simulink model "mesh"  (R2015a)
settings: Solver=ode45  StartTime=0.0  StopTime=10.0  RelTol=1e-3
libraries: fl_lib x7, nesl_utility x3
settings Model: SimulationMode=external  Creator=ASUS  LastModifiedBy=ASUS

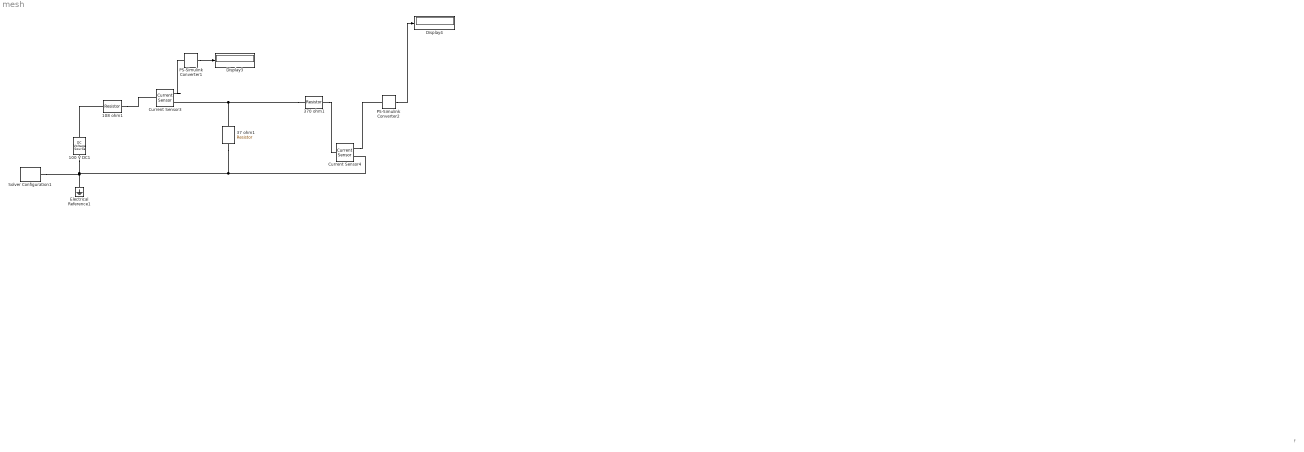
== system mesh ==
  note: f
  " 37 ohm1" : fl_lib/Electrical/Electrical Elements/Resistor  R=37 Ohm  i_specify=off  i_priority=High  i=0 A  v_specify=off  v_priority=High  v=0 V
  100 V DC1 : fl_lib/Electrical/Electrical Sources/DC Voltage Source  v0=100 V
  108 ohm1 : fl_lib/Electrical/Electrical Elements/Resistor  R=108 Ohm  i_specify=off  i_priority=High  i=0 A  v_specify=off  v_priority=High  v=0 V
  370 ohm1 : fl_lib/Electrical/Electrical Elements/Resistor  R=370 Ohm  i_specify=off  i_priority=High  i=0 A  v_specify=off  v_priority=High  v=0 V
  Current Sensor3 : fl_lib/Electrical/Electrical Sensors/Current Sensor
  Current Sensor4 : fl_lib/Electrical/Electrical Sensors/Current Sensor
  Display3 : Display
  Display4 : Display
  Electrical Reference1 : fl_lib/Electrical/Electrical Elements/Electrical Reference
  PS-Simulink Converter1 : nesl_utility/PS-Simulink Converter  PhysicalDomain=network_engine_domain  SubClassName=ps_output  LeftPortType=input  RightPortType=output  PseudoPeriodic=off  Frequencies=[]  Unit=1  AffineConversion=off
  PS-Simulink Converter2 : nesl_utility/PS-Simulink Converter  PhysicalDomain=network_engine_domain  SubClassName=ps_output  LeftPortType=input  RightPortType=output  PseudoPeriodic=off  Frequencies=[]  Unit=1  AffineConversion=off
  Solver Configuration1 : nesl_utility/Solver Configuration  PhysicalDomain=network_engine_domain  SubClassName=solver  LeftPortType=input  RightPortType=generic  Accelerate=off  Tones=[]  Harmonics=[]  SimulateNoise=off  Profile=off  UseLocalSampling=off  EnableSwitchedLinearOptims=on  FrequencyDomain=off  UseCCode=off  RelTol=0.001  AbsTol=1e-06  MinStep=1e-09  ToWorkspace=off  RevertToSquareIcSolve=off  NumHomotopyIterations=100  DoDC=off  ResidualTolerance=1e-09  UseLocalSolver=off  LocalSolverChoice=NE_BACKWARD_EULER_ADVANCER  LocalSolverSampleTime=0.001  DoFixedCost=off  MaxNonlinIter=3  MaxModeIter=2  LinearAlgebra=Sparse  DelaysMemoryBudget=1024  AutomaticFiltering=on  FilteringTimeConstant=0.001
  wires:
  PS-Simulink Converter1/1 -> Display3/1
  PS-Simulink Converter2/1 -> Display4/1
  connections:
  370 ohm1/LConn1 -- Current Sensor3/RConn2 -- " 37 ohm1"/LConn1
  Current Sensor4/RConn2 -- Solver Configuration1/RConn1 -- Electrical Reference1/LConn1 -- 100 V DC1/RConn1 -- " 37 ohm1"/RConn1
  370 ohm1/RConn1 -- Current Sensor4/LConn1
  100 V DC1/LConn1 -- 108 ohm1/LConn1
  108 ohm1/RConn1 -- Current Sensor3/LConn1
  Current Sensor3/RConn1 -- PS-Simulink Converter1/LConn1
  Current Sensor4/RConn1 -- PS-Simulink Converter2/LConn1
